simulink model "Elevator"  (R2024a)
settings: Solver=VariableStepAuto  StartTime=0.0  StopTime=inf  RelTol=1e-3
settings Model: Creator=Lenovo  LastModifiedBy=Lenovo

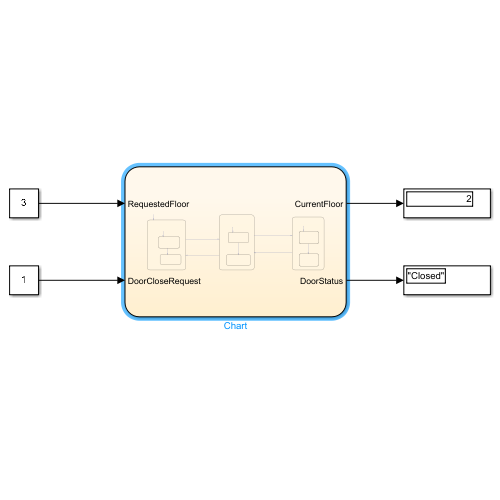
[thumbnail: Simulink's stored preview of the top-level diagram]
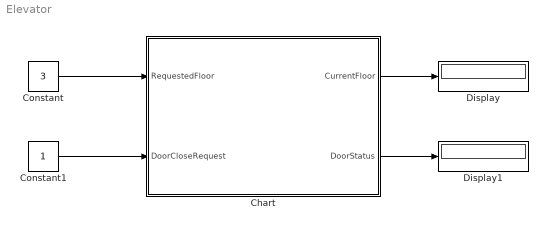
== system Elevator ==
  Chart : Stateflow chart  TreatAsAtomicUnit=on
  Constant : Constant  Value=3
  Constant1 : Constant
  Display : Display
  Display1 : Display
  wires:
  Constant1/1 -> Chart/2(DoorCloseRequest)
  Constant/1 -> Chart/1(RequestedFloor)
  Chart/1(CurrentFloor) -> Display/1
  Chart/2(DoorStatus) -> Display1/1

== stateflow chart Elevator/Chart ==
  state floor2
    entry:
    CurrentFloor = 2;
    state dooropened
      entry:
      DoorStatus = "Open";
    state doorclosed
      entry:
      DoorStatus = "Closed";
    (default) -> floor2.dooropened
    floor2.dooropened -> floor2.doorclosed : [DoorCloseRequest]
  state floor3
    entry:
    CurrentFloor = 3;
    state dooropened
      entry:
      DoorStatus = "Open";
    state doorclosed
      entry:
      DoorStatus = "Closed";
    (default) -> floor3.dooropened
    floor3.dooropened -> floor3.doorclosed : [DoorCloseRequest]
  state floor1
    entry:
    CurrentFloor = 1;
    state dooropened
      entry:
      DoorStatus = "Open";
    state doorclosed
      entry:
      DoorStatus = "Closed";
    (default) -> floor1.dooropened
    floor1.dooropened -> floor1.doorclosed : [DoorCloseRequest]
  (default) -> floor1
  floor2 -> floor3 [order 2] : [RequestedFloor == 3 &&...
      | DoorStatus=="Closed"]
  floor1 -> floor2 : [RequestedFloor ~= 1 &&...
      | DoorStatus=="Closed"]
  floor2 -> floor1 [order 1] : [RequestedFloor == 1 &&...
      | DoorStatus == "Closed"]
  floor3 -> floor2 : [RequestedFloor == 2 &&...
      | DoorStatus == "Closed"]
  data: RequestedFloor input; CurrentFloor output; DoorCloseRequest input; DoorStatus output string
